simulink model "resonator"  (R2018b)
settings: Solver=ode23s  StartTime=0.0  StopTime=5e-3  MaxStep=1e-4  RelTol=1e-3
values from neighbouring files (symbols this model uses):
  Ctuning = Cts(IV)    [line_par_resonator.m]
  tsim = 1/frq(IV)*1000    [line_par_resonator.m]
undefined symbols (not defined in the file or in its folder): C150, C150S, C230, Cf1, Cf2, L150, L150S, L230, Lf1, Lf2, R150, R150S, R230, Rf1, Rf2
libraries: powerlib x27, powerlib_meascontrol x1
settings Model: Creator=gasparini  LastModifiedBy=Riccardo
settings DebuggingCC: UnconnectedInputMsg=none  UnconnectedOutputMsg=none  UnconnectedLineMsg=none
settings SFSimCC: SimUseLocalCustomCode=off
settings RTWCC: RTWUseLocalCustomCode=off

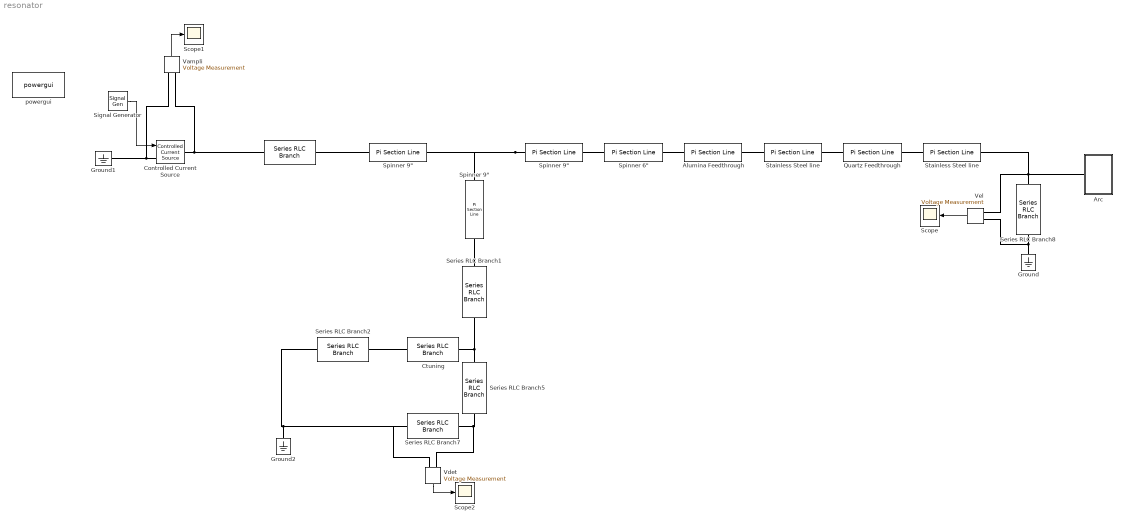
== system resonator ==
  " " : powerlib/Elements/Series RLC Branch  LConnTagsString=__new0  RConnTagsString=__new0  BranchType=C  Resistance=1  Inductance=3.6e-6  SetiL0=off  InitialCurrent=0  Capacitance=2500*1e-12  Setx0=off  InitialVoltage=0  Measurements=None
      settings: SourceProductName=Simscape Electrical
  "Alumina Feedthrough " : powerlib/Elements/Pi Section Line  LConnTagsString=__new0  RConnTagsString=__new0  Frequency=50e6  Resistance=Rf1*1e3  Inductance=Lf1*1e3  Capacitance=Cf1*1e3  Length=0.02e-3  PiSections=5  Measurements=None
      settings: AttributesFormatString=\n  SourceProductName=Simscape Electrical  SourceProductBaseCode=PS
  Arc : Subsystem
  Controlled Current Source : powerlib/Electrical Sources/Controlled Current Source  Initialize=on  Source_Type=AC  Amplitude=0  Phase=0  Frequency=0  Measurements=None
      settings: SourceProductName=Simscape Electrical
  Ctuning : powerlib/Elements/Series RLC Branch  LConnTagsString=__new0  RConnTagsString=__new0  BranchType=C  Resistance=1  Inductance=3.6e-6  SetiL0=off  InitialCurrent=0  Capacitance=Ctuning  Setx0=off  InitialVoltage=0  Measurements=None
      settings: SourceProductName=Simscape Electrical
  Ground : powerlib/Elements/Ground  LConnTagsString=a
      settings: SourceProductName=Simscape Electrical
  Ground1 : powerlib/Elements/Ground  LConnTagsString=a
      settings: SourceProductName=Simscape Electrical
  Ground2 : powerlib/Elements/Ground  LConnTagsString=a
      settings: SourceProductName=Simscape Electrical
  Quartz Feedthrough : powerlib/Elements/Pi Section Line  LConnTagsString=__new0  RConnTagsString=__new0  Frequency=50e6  Resistance=Rf2*1e3  Inductance=Lf2*1e3  Capacitance=Cf2*1e3  Length=0.01e-3  PiSections=5  Measurements=None
      settings: AttributesFormatString=\n  SourceProductName=Simscape Electrical  SourceProductBaseCode=PS
  Scope : Scope
  Scope1 : Scope
  Scope2 : Scope
  Series RLC Branch1 : powerlib/Elements/Series RLC Branch  LConnTagsString=__new0  RConnTagsString=__new0  BranchType=L  Resistance=1  Inductance=1e-9  SetiL0=off  InitialCurrent=0  Capacitance=1e-6  Setx0=off  InitialVoltage=0  Measurements=None
      settings: SourceProductName=Simscape Electrical
  Series RLC Branch2 : powerlib/Elements/Series RLC Branch  LConnTagsString=__new0  RConnTagsString=__new0  BranchType=RL  Resistance=2e-3  Inductance=30e-9  SetiL0=off  InitialCurrent=0  Capacitance=1e-6  Setx0=off  InitialVoltage=0  Measurements=None
      settings: SourceProductName=Simscape Electrical
  Series RLC Branch5 : powerlib/Elements/Series RLC Branch  LConnTagsString=__new0  RConnTagsString=__new0  BranchType=L  Resistance=1  Inductance=250e-6  SetiL0=off  InitialCurrent=0  Capacitance=1e-6  Setx0=off  InitialVoltage=0  Measurements=None
      settings: SourceProductName=Simscape Electrical
  Series RLC Branch7 : powerlib/Elements/Series RLC Branch  LConnTagsString=__new0  RConnTagsString=__new0  BranchType=R  Resistance=50  Inductance=3.6e-6  SetiL0=off  InitialCurrent=0  Capacitance=3.3e-9  Setx0=off  InitialVoltage=0  Measurements=None
      settings: SourceProductName=Simscape Electrical
  Series RLC Branch8 : powerlib/Elements/Series RLC Branch  LConnTagsString=__new0  RConnTagsString=__new0  BranchType=C  Resistance=1  Inductance=3.6e-6  SetiL0=off  InitialCurrent=0  Capacitance=5e-12  Setx0=off  InitialVoltage=0  Measurements=None
      settings: SourceProductName=Simscape Electrical
  Signal Generator : SignalGenerator  Frequency=45231073.8847
  "Spinner 6\"" : powerlib/Elements/Pi Section Line  LConnTagsString=__new0  RConnTagsString=__new0  Frequency=50e6  Resistance=R150S*1e3  Inductance=L150S*1e3  Capacitance=C150S*1e3  Length=0.3e-3  PiSections=5  Measurements=None
      settings: AttributesFormatString=\n  SourceProductName=Simscape Electrical  SourceProductBaseCode=PS
  "Spinner 9\"" : powerlib/Elements/Pi Section Line  LConnTagsString=__new0  RConnTagsString=__new0  Frequency=50e6  Resistance=R230*1e3  Inductance=L230*1e3  Capacitance=C230*1e3  Length=0.4e-3  PiSections=5  Measurements=None
      settings: AttributesFormatString=\n  SourceProductName=Simscape Electrical  SourceProductBaseCode=PS
  "Spinner 9\" " : powerlib/Elements/Pi Section Line  LConnTagsString=__new0  RConnTagsString=__new0  Frequency=50e6  Resistance=R230*1e3  Inductance=L230*1e3  Capacitance=C230*1e3  Length=0.3e-3  PiSections=5  Measurements=None
      settings: AttributesFormatString=\n  SourceProductName=Simscape Electrical  SourceProductBaseCode=PS
  "Spinner 9\" " : powerlib/Elements/Pi Section Line  LConnTagsString=__new0  RConnTagsString=__new0  Frequency=50e6  Resistance=R230*1e3  Inductance=L230*1e3  Capacitance=C230*1e3  Length=0.3e-3  PiSections=5  Measurements=None
      settings: AttributesFormatString=\n  SourceProductName=Simscape Electrical  SourceProductBaseCode=PS
  Stainless Steel line : powerlib/Elements/Pi Section Line  LConnTagsString=__new0  RConnTagsString=__new0  Frequency=50e6  Resistance=R150*1e3  Inductance=L150*1e3  Capacitance=C150*1e3  Length=0.5e-3  PiSections=5  Measurements=None
      settings: AttributesFormatString=\n  SourceProductName=Simscape Electrical  SourceProductBaseCode=PS
  "Stainless Steel line " : powerlib/Elements/Pi Section Line  LConnTagsString=__new0  RConnTagsString=__new0  Frequency=50e6  Resistance=R150*1e3  Inductance=L150*1e3  Capacitance=C150*1e3  Length=0.4e-3  PiSections=5  Measurements=None
      settings: AttributesFormatString=\n  SourceProductName=Simscape Electrical  SourceProductBaseCode=PS
  Vampli : powerlib/Measurements/Voltage Measurement  PhasorSimulation=off  OutputType=Complex  PSBequivalent=0
      settings: SourceProductName=Simscape Electrical
  "Vdet " : powerlib/Measurements/Voltage Measurement  PhasorSimulation=off  OutputType=Complex  PSBequivalent=0
      settings: SourceProductName=Simscape Electrical
  Vel : powerlib/Measurements/Voltage Measurement  PhasorSimulation=off  OutputType=Complex  PSBequivalent=0
      settings: SourceProductName=Simscape Electrical
  powergui : powerlib/powergui  Priority=1  SimulationMode=Continuous  SampleTime=50e-6  frequency=60  Iterations=50  frequencyindice=0  Pbase=100e6  ErrMax=1e-4  UnitsV=kV  UnitsW=MW  buscounter=0  FunctionMessages=off  echomessages=off  EnableUseOfTLC=off  CurrentSourceSwitches=off  DisableSnubberDevices=off  DisableRonSwitches=off  DisableVfSwitches=off  DisplayEquations=off  SolverType=Tustin/Backward Euler (TBE)  Interpol=off  ExternalGateDelay=off  methode=off  Ts=100  x0status=blocks  SPID=on  SwTol=0  HookPort=off  RestoreLinks=warning  ResistiveCurrentMeasurement=off  Frange=[30e6:0.1e4:60e6]  Ylog=on  Xlog=off  ShowGrid=on  save=off  variable=ZData  structure=0  ZoomFFT=off  StartTime=0.0  cycles=1  DisplayStyle=1  fundamental=60  FreqAxis=off  MaxFrequency=1000  frequencyindicesteady=1  RmsSteady=1  display=off
  wires:
  Vel/1 -> Scope/1
  Vampli/1 -> Scope1/1
  "Vdet "/1 -> Scope2/1
  Signal Generator/1 -> Controlled Current Source/1
  connections:
  "Spinner 9\""/LConn1 -- "Spinner 9\" "/LConn1 -- "Spinner 9\" "/RConn1
  "Spinner 6\""/LConn1 -- "Spinner 9\""/RConn1
  "Stainless Steel line "/LConn1 -- "Alumina Feedthrough "/RConn1
  " "/LConn1 -- "Spinner 9\" "/LConn1
  Controlled Current Source/LConn1 -- Ground1/LConn1 -- Vampli/LConn2
  Series RLC Branch7/LConn1 -- "Vdet "/LConn2 -- Series RLC Branch5/RConn1
  Ctuning/LConn1 -- Series RLC Branch1/RConn1 -- Series RLC Branch5/LConn1
  Series RLC Branch8/LConn1 -- Arc/LConn1 -- Stainless Steel line/RConn1 -- Vel/LConn1
  "Spinner 6\""/RConn1 -- "Alumina Feedthrough "/LConn1
  Vel/LConn2 -- Ground/LConn1 -- Series RLC Branch8/RConn1
  "Spinner 9\" "/RConn1 -- Series RLC Branch1/LConn1
  Quartz Feedthrough/RConn1 -- Stainless Steel line/LConn1
  Quartz Feedthrough/LConn1 -- "Stainless Steel line "/RConn1
  Series RLC Branch2/LConn1 -- Ctuning/RConn1
  Ground2/LConn1 -- "Vdet "/LConn1 -- Series RLC Branch7/RConn1 -- Series RLC Branch2/RConn1
  " "/RConn1 -- Controlled Current Source/RConn1 -- Vampli/LConn1

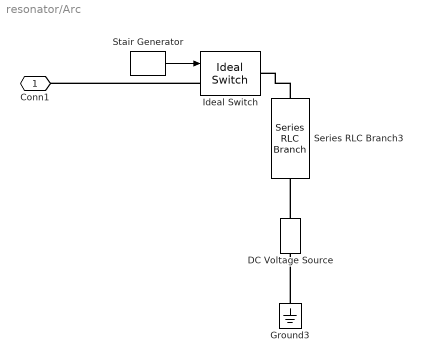
== system resonator/Arc ==
  DC Voltage Source : powerlib/Electrical Sources/DC Voltage Source  Amplitude=20  Measurements=None
  Ground3 : powerlib/Elements/Ground  LConnTagsString=a
      settings: SourceProductName=Simscape Electrical
  Ideal Switch : powerlib/Power Electronics/Ideal Switch  Ron=0.001  Lon=0  IC=0  Rs=1e5  Cs=inf  Measurements=off
  Series RLC Branch3 : powerlib/Elements/Series RLC Branch  LConnTagsString=__new0  RConnTagsString=__new0  BranchType=L  Resistance=1  Inductance=20e-9  SetiL0=off  InitialCurrent=0  Capacitance=1e-6  Setx0=off  InitialVoltage=0  Measurements=None
      settings: SourceProductName=Simscape Electrical
  Stair Generator : powerlib_meascontrol/Pulse & Signal Generators/Stair Generator  t=[0.7*tsim]  e=[1]  Ts=0
      settings: SourceProductName=Simscape Electrical
  Conn1 : PMIOPort  Side=Left
  wires:
  Stair Generator/1 -> Ideal Switch/1
  connections:
  DC Voltage Source/RConn1 -- Series RLC Branch3/RConn1
  Ideal Switch/LConn1 -- Conn1/RConn1
  Series RLC Branch3/LConn1 -- Ideal Switch/RConn1
  Ground3/LConn1 -- DC Voltage Source/LConn1
